simulink library "FindCoMPosition_ul"  (R2018a)
settings: Solver=VariableStepAuto  StartTime=0.0  StopTime=10.0  RelTol=1e-3
settings Model: Creator=mcobb  LastModifiedBy=mcobb

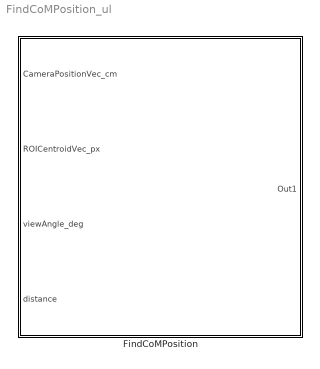
== system FindCoMPosition_ul ==
  FindCoMPosition : Subsystem

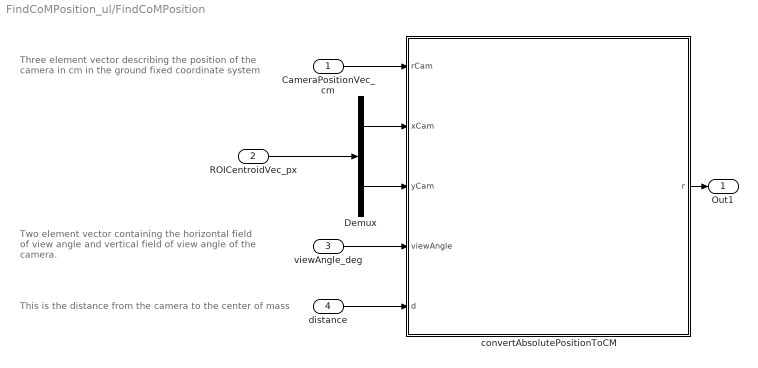
== system FindCoMPosition_ul/FindCoMPosition ==
  note: Three element vector describing the position of the
      | camera in cm in the ground fixed coordinate system
  note: This is the distance from the camera to the center of mass
  note: Two element vector containing the horizontal
      | field of view angle and vertical field of view angle
      | of the camera.
  CameraPositionVec_cm : Inport
  ROICentroidVec_px : Inport  Port=2
  viewAngle_deg : Inport  Port=3
  distance : Inport  Port=4
  Demux : Demux  Outputs=2
  convertAbsolutePositionToCM : MATLAB Function  TreatAsAtomicUnit=on
  Out1 : Outport
  wires:
  CameraPositionVec_cm/1 -> convertAbsolutePositionToCM/1(rCam)
  viewAngle_deg/1 -> convertAbsolutePositionToCM/4(viewAngle)
  distance/1 -> convertAbsolutePositionToCM/5(d)
  convertAbsolutePositionToCM/1(r) -> Out1/1
  ROICentroidVec_px/1 -> Demux/1
  Demux/1 -> convertAbsolutePositionToCM/2(xCam)
  Demux/2 -> convertAbsolutePositionToCM/3(yCam)

== matlab function FindCoMPosition_ul/FindCoMPosition/convertAbsolutePositionToCM ==
  data: rCam input; xCam input; yCam input; viewAngle input; d input; r output size=[1 3]
function r = convertAbsolutePositionsToCM(rCam, xCam, yCam,  viewAngle, d)
%#codegen
% This function calculates the x, y and z position of the dots in the
% ground fixed coordinates

% INPUTS
% rCam - 3 element vector of the camera position in the ground fixed frame
% units:cm
% xCam - horitontal location of the dots centroid in the image frame
% units:pixels
% yCam - vertical location of the dots centroid in the image frame
% units:pixels
% viewAngle - two element vector, first characterizes the width of the
% field of view (camera horizontal), the second characterizes the height of
% the field of veiw (camera vertical).
% d - distance from the camera to the dots

% Calculate the x and y locations
% If the horizontal location of the dots centroid in the image frame is
% to the left of the centerline (xCam<1020) then the y position of the dots
% centroid in the ground fixed frame will be less than the y position of
% the camera in the ground fixed frame.
% If the vertical location of the dots centroid in the image frame is
% below the centerline (yCam>544) then the x position of the dots
% centroid in the ground fixed frame will be greater than the x position of
% the camera in the ground fixed frame.
% d=50;

x = rCam(1) + (yCam - 544 )*((2*d*tand(viewAngle(1)))/1088);
y = rCam(2) + (xCam - 1020)*((2*d*tand(viewAngle(2)))/2040);

% Calculate the z coordinate of the centroid of the dots.
% We know the x and y coordinate, the position of the camera, and the
% distance fromt the cammera to the dots.  Therfore, the solution is the
% value of z which causes the position to lie on the sphere centered on the
% camera with radius = d
z = 0;
% Check first to make sure that the value under the sqrt is positive
if d^2-(x - rCam(1))^2-(y - rCam(2))^2>=0
    z  = rCam(3) + sqrt(d^2-(x - rCam(1))^2-(y - rCam(2))^2);
end

r  =  [x y z];
